simulink model "UdpSigSocket_Complete"  (R2013a)
settings: Solver=ode1  StartTime=0.0  StopTime=inf  FixedStep=0.04  RelTol=1e-3
StartFcn:
  | close all
settings Model: Creator=jsUni  LastModifiedBy=jsUni
settings DataIOCC: SignalLoggingSaveFormat=ModelDataLogs
settings DebuggingCC: MultiTaskDSMMsg=warning  MultiTaskCondExecSysMsg=none  StrictBusMsg=None
settings RTWCC: IncludeERTFirstTime=on

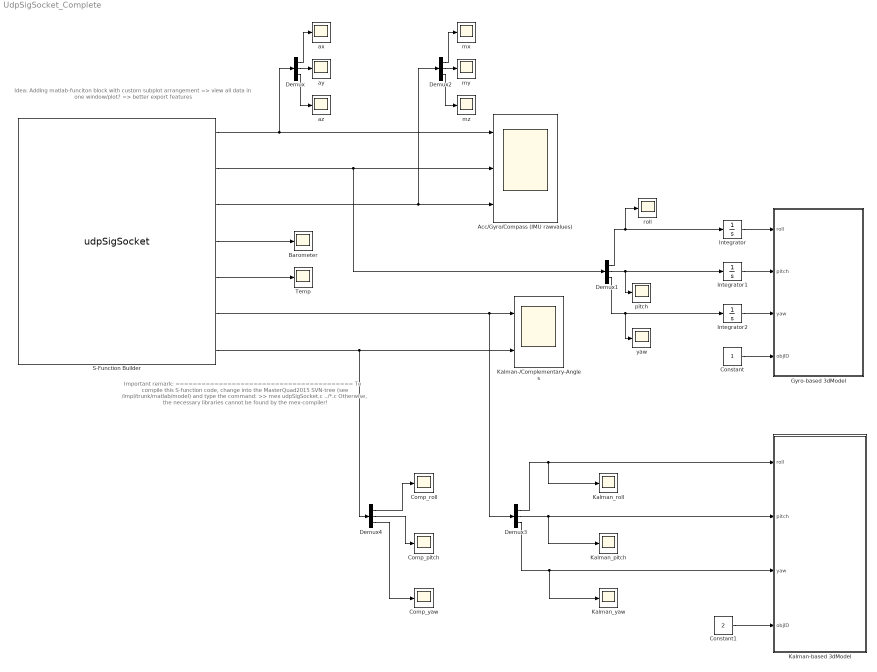
== system UdpSigSocket_Complete ==
  note: Important remark:
      | =========================================
      |  To compile this S-function code, change into the MasterQuad2015
      | SVN-tree (see /impl/trunk/matlab/model) and type the command:
      | >> mex udpSigSocket.c ../*.c
      |
      | Otherwise, the necessary libraries cannot be found by the mex-compiler!
  note: Idea:
      | Adding matlab-funciton block with custom
      | subplot arrangement
      | => view all data in one window/plot? => better export features
  Acc/Gyro/Compass (IMU rawvalues) : Scope  NumInputPorts=3
      settings: YMin=-11~-35~-1e-06  YMax=1~15~1e-05
  Barometer : Scope
      settings: YMin=989.08  YMax=989.22  SaveName=ScopeData3
  Comp_pitch : Scope
      settings: ShowLegends=on  TimeRange=1000  YMin=-45  YMax=15  SaveName=Comp_pitch
  Comp_roll : Scope
      settings: TimeRange=1000  YMin=-0.5025  YMax=-0.4625  SaveName=Comp_roll
  Comp_yaw : Scope
      settings: TimeRange=1000  YMin=78.525  YMax=78.95  SaveName=Comp_yaw
  Constant : Constant
  Constant1 : Constant  Value=2
  Demux{,1..4} (5 alike) : Demux  Outputs=3
  Gyro-based 3dModel : MATLAB Function  TreatAsAtomicUnit=on
  Integrator : Integrator
  Integrator1 : Integrator
  Integrator2 : Integrator
  Kalman-/Complementary-Angles : Scope  NumInputPorts=2
      settings: ShowLegends=on  TimeRange=2000  YMin=-175~-175  YMax=150~150  SaveName=ScopeData5
  Kalman-based 3dModel : MATLAB Function  TreatAsAtomicUnit=on
  Kalman_pitch : Scope
      settings: ShowLegends=on  TimeRange=1000  YMin=-85  YMax=0  SaveName=Kalman_pitch
  Kalman_roll : Scope
      settings: TimeRange=1000  YMin=0  YMax=85  SaveName=Kalman_roll
  Kalman_yaw : Scope
      settings: TimeRange=1000  YMin=-110  YMax=20  SaveName=Kalman_yaw
  S-Function Builder : S-Function  InitFcn=try, set_param(gcb,'FunctionName','udpSigSocket'), end  FunctionName=udpSigSocket  Parameters=0.04,5000  SFunctionModules=udpSigSocket_wrapper  EnableBusSupport=off  mask(S-Function Builder){}
      mask help: Simulink:masks:SFunctionBuilder_MD
      mask init:
      | val = [[.9  0.75 0.75 1 1 .9 .9 1]',[1 1 0.75 0.75 .9 .9 1 .9]'];try , sys = get_param(gcb,'SfunBuilderFcnName');if isempty(sys), sys = get_param(gcb,'FunctionName'); end,catch, sys = get_param(gcb,'FunctionName'); end
      settings: CopyFcn=set_param(gcbh,'LinkStatus','none')  PreSaveFcn=try, set_param(gcb,'FunctionName','udpSigSocket'), end  OpenFcn=sfunctionwizard(gcbh)
      mask Display: plot(val(:,1),val(:,2)),disp(sys), port_label('output',1,'Raw_Accelerometer_xyz'), port_label('output',2,'Raw_Gyrometer_rpy'), port_label('output',3,'Raw_Compass_xyz'), port_label('output',4,'Raw_Barometer_z'), port_label('output',5,'Raw_Temperature'), port_label('output',6,'Kalman_Angles_rpy'), port_label('output',7,'Complementary_Angles_rpy')
  Temp : Scope
      settings: YMin=32.2  YMax=32.29  SaveName=ScopeData4
  ax : Scope
      settings: YMin=-0.275  YMax=0.125  SaveName=ax
  ay : Scope
      settings: ShowLegends=on  YMin=-9.575  YMax=-9.3  SaveName=ay
  az : Scope
      settings: YMin=-10.8  YMax=-9.85  SaveName=az
  mx : Scope
      settings: TimeRange=1000  YMin=-2e-05  YMax=2.5e-05  SaveName=mx
  my : Scope
      settings: ShowLegends=on  TimeRange=1000  YMin=-2e-05  YMax=2.5e-05  SaveName=my
  mz : Scope
      settings: TimeRange=1000  YMin=-1.5e-05  YMax=2.5e-05  SaveName=mz
  pitch : Scope
      settings: ShowLegends=on  TimeRange=1000  YMin=-10  YMax=15  SaveName=pitch
  roll : Scope
      settings: TimeRange=1000  YMin=-100  YMax=50  SaveName=roll
  yaw : Scope
      settings: TimeRange=1000  YMin=-90  YMax=80  SaveName=yaw
  wires:
  S-Function Builder/3 -> Demux2/1, Acc/Gyro/Compass (IMU rawvalues)/3
  S-Function Builder/2 -> Demux1/1, Acc/Gyro/Compass (IMU rawvalues)/2
  S-Function Builder/1 -> Demux/1, Acc/Gyro/Compass (IMU rawvalues)/1
  S-Function Builder/5 -> Temp/1
  S-Function Builder/4 -> Barometer/1
  S-Function Builder/7 -> Kalman-/Complementary-Angles/2, Demux4/1
  Demux/1 -> ax/1
  Demux/2 -> ay/1
  Demux/3 -> az/1
  Demux1/1 -> roll/1, Integrator/1
  Demux1/2 -> pitch/1, Integrator1/1
  Demux1/3 -> Integrator2/1, yaw/1
  Demux2/1 -> mx/1
  Demux2/2 -> my/1
  Demux2/3 -> mz/1
  S-Function Builder/6 -> Demux3/1, Kalman-/Complementary-Angles/1
  Demux3/1 -> Kalman-based 3dModel/1(roll), Kalman_roll/1
  Demux3/2 -> Kalman_pitch/1, Kalman-based 3dModel/2(pitch)
  Demux4/1 -> Comp_roll/1
  Demux4/2 -> Comp_pitch/1
  Demux4/3 -> Comp_yaw/1
  Demux3/3 -> Kalman_yaw/1, Kalman-based 3dModel/3(yaw)
  Integrator/1 -> Gyro-based 3dModel/1(roll)
  Integrator1/1 -> Gyro-based 3dModel/2(pitch)
  Integrator2/1 -> Gyro-based 3dModel/3(yaw)
  Constant/1 -> Gyro-based 3dModel/4(objID)
  Constant1/1 -> Kalman-based 3dModel/4(objID)

== matlab function UdpSigSocket_Complete/Gyro-based 3dModel ==
  data: roll input; pitch input; yaw input; objID input
function drawBox ( roll, pitch,yaw, objID)
coder.extrinsic('patch');
coder.extrinsic('set');

persistent figureArray patchArray crossArray;

x1 = [-2 -2 2 2 -2]; 
y1 = [-4 4 4 -4 -4]; 
z1 = [0 0 0 0 0 ]; 

xx = [0 1]; 
yx = [0 0]; 
zx = [0 0];

xy = [0 0]; 
yy = [0 1]; 
zy = [0 0];

xz = [0 0]; 
yz = [0 0]; 
zz = [0 1];

if isempty(figureArray)
    objIDMax=2;
    figureArray=zeros(objIDMax,1);
    figureArray(objID) = figure;
    
    patchArray=zeros(objIDMax,1);
    patchArray(objID) = patch(x1, y1, z1,'r');

    crossArray = zeros(objIDMax,3);
    hold on
    crossArray(objID,1) = plot3(xx,yx,zx,'k','LineWidth',2); %x
    crossArray(objID,2) = plot3(xy,yy,zy,'k','LineWidth',2); %y
    crossArray(objID,3) = plot3(zx,zy,zz,'k','LineWidth',2); %z
        
    xlabel('x'); ylabel('y'); zlabel('z');
    if (objID == 1)
        title('Raw gyro sensors (integrated)');
    else
        title('Filtered (RPi output)');
    end
    grid
    axis([-7 7 -7 7 -7 7])
    view([45 15])
end

Rroll = [1,0,0;
         0, cosd(roll), -sind(roll);
         0, sind(roll), cosd(roll)];
Rpitch = [cosd(pitch),0,sind(pitch);
         0,1,0;
         -sind(pitch),0, cosd(pitch)];
Ryaw = [ cosd(yaw), -sind(yaw),0;
         sind(yaw), cosd(yaw),0;
         0,0,1];

xRot=zeros(size(x1));
yRot=zeros(size(y1));
zRot=zeros(size(z1));
for i=1:length(xRot)
    temp=Rroll*Rpitch*Ryaw*[x1(i);y1(i);z1(i)];
    xRot(i)=temp(1);
    yRot(i)=temp(2);
    zRot(i)=temp(3);
end

xxRot=zeros(size(xx));
yxRot=zeros(size(yx));
zxRot=zeros(size(zx));
for i=1:length(xxRot)
    temp=Rroll*Rpitch*Ryaw*[xx(i);yx(i);zx(i)];
    xxRot(i)=temp(1);
    yxRot(i)=temp(2);
    zxRot(i)=temp(3);
end
set(crossArray( objID,1), 'XData', xxRot);
set(crossArray( objID,1), 'YData', yxRot);
set(crossArray( objID,1), 'ZData', zxRot);

xyRot=zeros(size(xy));
yyRot=zeros(size(yy));
zyRot=zeros(size(zy));
for i=1:length(xyRot)
    temp=Rroll*Rpitch*Ryaw*[xy(i);yy(i);zy(i)];
    xyRot(i)=temp(1);
    yyRot(i)=temp(2);
    zyRot(i)=temp(3);
end
set(crossArray( objID,2), 'XData', xyRot);
set(crossArray( objID,2), 'YData', yyRot);
set(crossArray( objID,2), 'ZData', zyRot);


xzRot=zeros(size(xz));
yzRot=zeros(size(yz));
zzRot=zeros(size(zz));
for i=1:length(xzRot)
    temp=Rroll*Rpitch*Ryaw*[xz(i);yz(i);zz(i)];
    xzRot(i)=temp(1);
    yzRot(i)=temp(2);
    zzRot(i)=temp(3);
end
set(crossArray( objID,3), 'XData', xzRot);
set(crossArray( objID,3), 'YData', yzRot);
set(crossArray( objID,3), 'ZData', zzRot);


set(patchArray( objID ),'XData', xRot);
set(patchArray( objID ),'YData', yRot);
set(patchArray( objID ),'ZData', zRot);
drawnow
end

== matlab function UdpSigSocket_Complete/Kalman-based 3dModel ==
  data: roll input; pitch input; yaw input; objID input
function drawBox ( roll, pitch,yaw, objID)
coder.extrinsic('patch');
coder.extrinsic('set');

persistent figureArray patchArray crossArray;

x1 = [-2 -2 2 2 -2]; 
y1 = [-4 4 4 -4 -4]; 
z1 = [0 0 0 0 0 ]; 

xx = [0 1]; 
yx = [0 0]; 
zx = [0 0];

xy = [0 0]; 
yy = [0 1]; 
zy = [0 0];

xz = [0 0]; 
yz = [0 0]; 
zz = [0 1];

if isempty(figureArray)
    objIDMax=2;
    figureArray=zeros(objIDMax,1);
    figureArray(objID) = figure;
    
    patchArray=zeros(objIDMax,1);
    patchArray(objID) = patch(x1, y1, z1,'g');

    crossArray = zeros(objIDMax,3);
    hold on
    crossArray(objID,1) = plot3(xx,yx,zx,'k','LineWidth',2); %x
    crossArray(objID,2) = plot3(xy,yy,zy,'k','LineWidth',2); %y
    crossArray(objID,3) = plot3(zx,zy,zz,'k','LineWidth',2); %z
        
    xlabel('x'); ylabel('y'); zlabel('z');
    if (objID == 1)
        title('Raw gyro sensors (integrated)');
    else
        title('Filtered (RPi output)');
    end
    grid
    axis([-7 7 -7 7 -7 7])
    view([45 15])
end

Rroll = [1,0,0;
         0, cosd(roll), -sind(roll);
         0, sind(roll), cosd(roll)];
Rpitch = [cosd(pitch),0,sind(pitch);
         0,1,0;
         -sind(pitch),0, cosd(pitch)];
Ryaw = [ cosd(yaw), -sind(yaw),0;
         sind(yaw), cosd(yaw),0;
         0,0,1];

xRot=zeros(size(x1));
yRot=zeros(size(y1));
zRot=zeros(size(z1));
for i=1:length(xRot)
    temp=Rroll*Rpitch*Ryaw*[x1(i);y1(i);z1(i)];
    xRot(i)=temp(1);
    yRot(i)=temp(2);
    zRot(i)=temp(3);
end

xxRot=zeros(size(xx));
yxRot=zeros(size(yx));
zxRot=zeros(size(zx));
for i=1:length(xxRot)
    temp=Rroll*Rpitch*Ryaw*[xx(i);yx(i);zx(i)];
    xxRot(i)=temp(1);
    yxRot(i)=temp(2);
    zxRot(i)=temp(3);
end
set(crossArray( objID,1), 'XData', xxRot);
set(crossArray( objID,1), 'YData', yxRot);
set(crossArray( objID,1), 'ZData', zxRot);

xyRot=zeros(size(xy));
yyRot=zeros(size(yy));
zyRot=zeros(size(zy));
for i=1:length(xyRot)
    temp=Rroll*Rpitch*Ryaw*[xy(i);yy(i);zy(i)];
    xyRot(i)=temp(1);
    yyRot(i)=temp(2);
    zyRot(i)=temp(3);
end
set(crossArray( objID,2), 'XData', xyRot);
set(crossArray( objID,2), 'YData', yyRot);
set(crossArray( objID,2), 'ZData', zyRot);


xzRot=zeros(size(xz));
yzRot=zeros(size(yz));
zzRot=zeros(size(zz));
for i=1:length(xzRot)
    temp=Rroll*Rpitch*Ryaw*[xz(i);yz(i);zz(i)];
    xzRot(i)=temp(1);
    yzRot(i)=temp(2);
    zzRot(i)=temp(3);
end
set(crossArray( objID,3), 'XData', xzRot);
set(crossArray( objID,3), 'YData', yzRot);
set(crossArray( objID,3), 'ZData', zzRot);


set(patchArray( objID ),'XData', xRot);
set(patchArray( objID ),'YData', yRot);
set(patchArray( objID ),'ZData', zRot);
drawnow
end
